simulink library "Springs_Axle2_Decoupled"  (R2026a)
settings: Solver=VariableStepAuto
libraries: Spring_Basics x6, fl_lib x4
Description:
  | Component of Simscape Vehicle Templates Library
  | 
  | Copyright 2018-2026 The MathWorks, Inc.
settings Model: Creator=smiller  LastModifiedBy=smiller

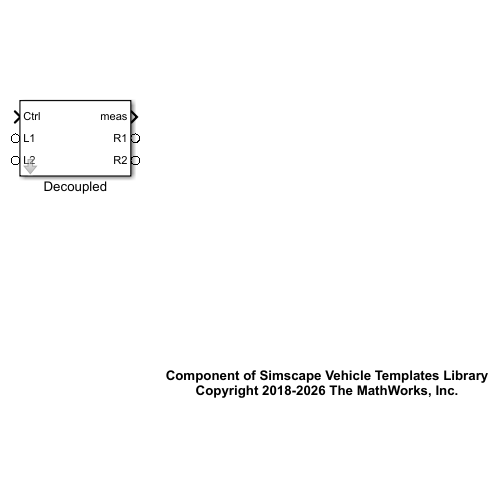
[thumbnail: Simulink's stored preview of the top-level diagram]
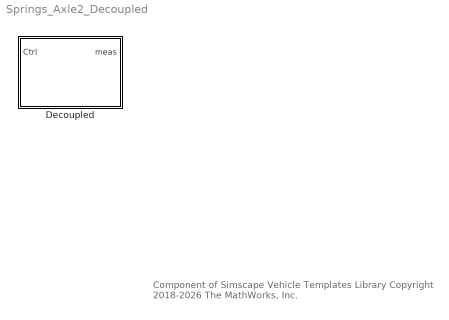
== system Springs_Axle2_Decoupled ==
  note: Component of Simscape Vehicle Templates Library
      | Copyright 2018-2026 The MathWorks, Inc.
  Decoupled : Subsystem  VariantControl=Independent  mask(Roll and Heave Springs){InitTriggerDropdown=0}
      mask prompts: InitTriggerDropdown "Initialization Trigger Dropdown"
      mask help: Models springs in a suspension design that decouples stiffness for body roll and heave .
      mask init:
      | curblk = gcb;
      | 
      | % Trigger Mask Initialization for 
      | % variant subsystems below this level
      | sm_car_lib_maskInitTrigger(curblk);
      mask TypeOptions InitTriggerDropdown: 0 | 1

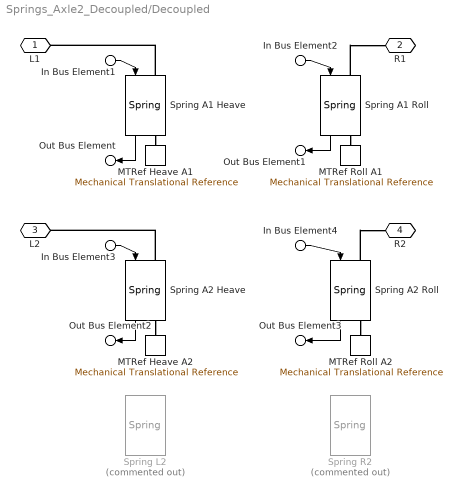
== system Springs_Axle2_Decoupled/Decoupled ==
  In Bus Element1 : Inport  PortName=Ctrl  Element=L1
  In Bus Element2 : Inport  PortName=Ctrl  Element=R1
  In Bus Element3 : Inport  PortName=Ctrl  Element=L2
  In Bus Element4 : Inport  PortName=Ctrl  Element=R2
  MTRef Heave A1 : fl_lib/Mechanical/Translational Elements/Mechanical Translational Reference
  MTRef Heave A2 : fl_lib/Mechanical/Translational Elements/Mechanical Translational Reference
  MTRef Roll A1 : fl_lib/Mechanical/Translational Elements/Mechanical Translational Reference
  MTRef Roll A2 : fl_lib/Mechanical/Translational Elements/Mechanical Translational Reference
  Spring A1 Heave : Spring_Basics/Spring  VariantControl=Variant1  LabelModeActiveChoice=Linear  Spring=Spring.Axle1.Heave  VariantLabel=Spring.Axle1.Heave.class.Value  InitTriggerDropdown=0
      settings: AttributesFormatString=%<ActiveVariant>
  Spring A1 Roll : Spring_Basics/Spring  VariantControl=Variant1  LabelModeActiveChoice=Linear  Spring=Spring.Axle1.Roll  VariantLabel=Spring.Axle1.Roll.class.Value  InitTriggerDropdown=0
      settings: AttributesFormatString=%<ActiveVariant>
  Spring A2 Heave : Spring_Basics/Spring  VariantControl=Variant1  LabelModeActiveChoice=Linear  Spring=Spring.Axle2.Heave  VariantLabel=Spring.Axle2.Heave.class.Value  InitTriggerDropdown=0
      settings: AttributesFormatString=%<ActiveVariant>
  Spring A2 Roll : Spring_Basics/Spring  VariantControl=Variant1  LabelModeActiveChoice=Linear  Spring=Spring.Axle2.Roll  VariantLabel=Spring.Axle2.Roll.class.Value  InitTriggerDropdown=0
      settings: AttributesFormatString=%<ActiveVariant>
  Spring L2 : Spring_Basics/Spring  Commented=on  VariantControl=Variant1  LabelModeActiveChoice=Linear  Spring=Spring.Axle2  VariantLabel=Spring.Axle2.class.Value  InitTriggerDropdown=0
      settings: AttributesFormatString=%<ActiveVariant>
  Spring R2 : Spring_Basics/Spring  Commented=on  VariantControl=Variant1  LabelModeActiveChoice=Linear  Spring=Spring.Axle2  VariantLabel=Spring.Axle2.class.Value  InitTriggerDropdown=0
      settings: AttributesFormatString=%<ActiveVariant>
  L1 : PMIOPort  Side=Left
  R1 : PMIOPort  Port=2  Side=Right
  L2 : PMIOPort  Port=3  Side=Left
  R2 : PMIOPort  Port=4  Side=Right
  Out Bus Element : Outport  VectorParamsAs1DForOutWhenUnconnected=off  PortName=meas  Element=L1
  Out Bus Element1 : Outport  VectorParamsAs1DForOutWhenUnconnected=off  PortName=meas  Element=R1
  Out Bus Element2 : Outport  VectorParamsAs1DForOutWhenUnconnected=off  PortName=meas  Element=L2
  Out Bus Element3 : Outport  VectorParamsAs1DForOutWhenUnconnected=off  PortName=meas  Element=R2
  wires:
  Spring A2 Roll/1 -> Out Bus Element3/1
  In Bus Element4/1 -> Spring A2 Roll/1
  Spring A2 Heave/1 -> Out Bus Element2/1
  In Bus Element3/1 -> Spring A2 Heave/1
  Spring A1 Roll/1 -> Out Bus Element1/1
  In Bus Element2/1 -> Spring A1 Roll/1
  Spring A1 Heave/1 -> Out Bus Element/1
  In Bus Element1/1 -> Spring A1 Heave/1
  connections:
  Spring A1 Heave/RConn1 -- MTRef Heave A1/LConn1
  Spring A1 Heave/LConn1 -- L1/RConn1
  Spring A2 Heave/RConn1 -- MTRef Heave A2/LConn1
  Spring A2 Heave/LConn1 -- L2/RConn1
  Spring A2 Roll/RConn1 -- MTRef Roll A2/LConn1
  Spring A2 Roll/LConn1 -- R2/RConn1
  Spring A1 Roll/RConn1 -- MTRef Roll A1/LConn1
  Spring A1 Roll/LConn1 -- R1/RConn1
